simulink model "robot_wheels"  (R2019b)
settings: Solver=VariableStepAuto  StartTime=0.0  StopTime=10.0  RelTol=1e-3
InitFcn:
  | L = 1;
  | x_ = 2;
  | y_ = 2;
  | Kv = 1;
  | Kt = 1;
model workspace (MAT data in the model file):
  Kt = 0.44604063924
  Kv = 1.77284659212
  L = 1
  x_ = -2
  y_ = -2
libraries: simulink x1
settings Model: OrderedModelArguments=off  Creator=Анастасия  LastModifiedBy=Анастасия

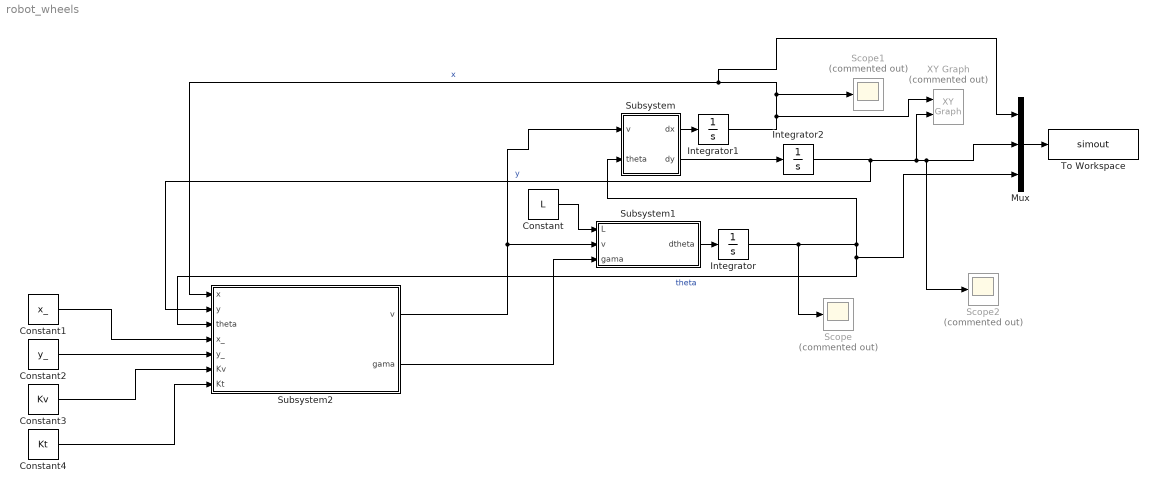
== system robot_wheels ==
  Constant : Constant  Value=L
  Constant1 : Constant  Value=x_
  Constant2 : Constant  Value=y_
  Constant3 : Constant  Value=Kv
  Constant4 : Constant  Value=Kt
  Integrator : Integrator
  Integrator1 : Integrator
  Integrator2 : Integrator
  Mux : Mux  Inputs=3
  Scope : Scope  Commented=on
  Scope1 : Scope  Commented=on
  Scope2 : Scope  Commented=on
  Subsystem : Subsystem
  Subsystem1 : Subsystem
  Subsystem2 : Subsystem
  To Workspace : ToWorkspace  VariableName=simout  SaveFormat=Timeseries  SampleTime=-1
  XY Graph : simulink/Sinks/XY Graph  Commented=on  xmin=-5  xmax=1  ymin=-5  ymax=1  st=-1
  wires:
  Subsystem2/1(v) -> Subsystem/1(v), Subsystem1/2(v)
  Subsystem1/1("dtheta ") -> Integrator/1
  Subsystem/1(dx) -> Integrator1/1
  Subsystem/2(dy) -> Integrator2/1
  Constant/1 -> Subsystem1/1(L)
  Subsystem2/2(gama) -> Subsystem1/3(gama)
  Mux/1 -> To Workspace/1
  Constant2/1 -> Subsystem2/5(y_)
  Constant1/1 -> Subsystem2/4(x_)
  Constant3/1 -> Subsystem2/6(Kv)
  Constant4/1 -> Subsystem2/7(Kt)
  Integrator/1 -> Scope/1, Subsystem/2(theta), Subsystem2/3(theta), Mux/3  "theta"
  Integrator1/1 -> XY Graph/1, Scope1/1, Subsystem2/1(x), Mux/1  "x"
  Integrator2/1 -> XY Graph/2, Scope2/1, Mux/2, Subsystem2/2(y)  "y"

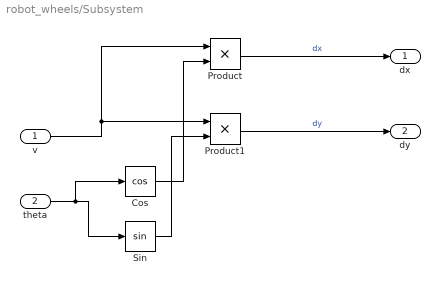
== system robot_wheels/Subsystem ==
  v : Inport
  theta : Inport  Port=2
  Cos : Trigonometry  Operator=cos
  Product : Product
  Product1 : Product
  Sin : Trigonometry
  dx : Outport
  dy : Outport  Port=2
  wires:
  v/1 -> Product1/1, Product/1
  Cos/1 -> Product/2
  theta/1 -> Cos/1, Sin/1
  Product/1 -> dx/1  "dx"
  Sin/1 -> Product1/2
  Product1/1 -> dy/1  "dy"

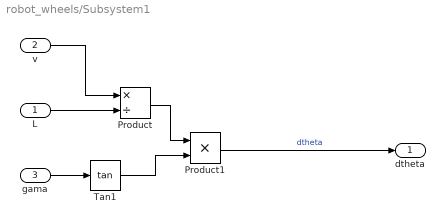
== system robot_wheels/Subsystem1 ==
  L : Inport
  v : Inport  Port=2
  gama : Inport  Port=3
  Product : Product  Inputs=*/
  Product1 : Product
  Tan1 : Trigonometry  Operator=tan
  "dtheta " : Outport
  wires:
  gama/1 -> Tan1/1
  v/1 -> Product/1
  L/1 -> Product/2
  Product/1 -> Product1/1
  Tan1/1 -> Product1/2
  Product1/1 -> "dtheta "/1  "dtheta"

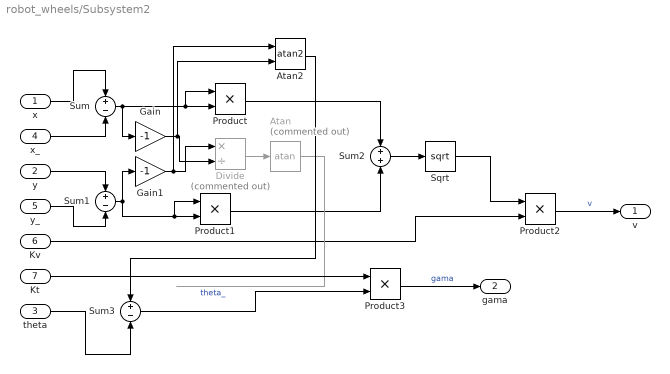
== system robot_wheels/Subsystem2 ==
  x : Inport
  y : Inport  Port=2
  theta : Inport  Port=3
  x_ : Inport  Port=4
  y_ : Inport  Port=5
  Kv : Inport  Port=6
  Kt : Inport  Port=7
  Atan : Trigonometry  Commented=on  Operator=atan
  Atan2 : Trigonometry  Operator=atan2
  Divide : Product  Commented=on  Inputs=*/
  Gain : Gain  Gain=-1
  Gain1 : Gain  Gain=-1
  Product{,1..3} (4 alike) : Product
  Sqrt : Sqrt  SaturateOnIntegerOverflow=on
  Sum : Sum  Inputs=+-
  Sum1 : Sum  Inputs=+-
  Sum2 : Sum
  Sum3 : Sum  Inputs=+-
  v : Outport
  gama : Outport  Port=2
  wires:
  x/1 -> Sum/1
  x_/1 -> Sum/2
  y/1 -> Sum1/1
  y_/1 -> Sum1/2
  Sum/1 -> Gain/1, Product/2, Product/1
  Sum1/1 -> Product1/1, Product1/2, Gain1/1
  Product/1 -> Sum2/1
  Product1/1 -> Sum2/2
  Sum2/1 -> Sqrt/1
  Kv/1 -> Product2/2
  Sqrt/1 -> Product2/1
  Product2/1 -> v/1  "v"
  Gain1/1 -> Atan2/1, Divide/1
  Gain/1 -> Atan2/2, Divide/2
  Divide/1 -> Atan/1
  Atan/1 -> ?  "theta_"
  theta/1 -> Sum3/2
  Kt/1 -> Product3/1
  Sum3/1 -> Product3/2
  Product3/1 -> gama/1  "gama"
  Atan2/1 -> Sum3/1
